simulink model "SoftRobot_AdaptivePassivity_FaultObserver_Regulation_S2"  (R2021b)
settings: Solver=FixedStepAuto  StartTime=0.0  StopTime=15  FixedStep=0.001  RelTol=1e-3  EnableMultiTasking=on
(part 1 of 2)
settings Model: Creator=Amirhosein  LastModifiedBy=sinar
settings SolverCC: AlgebraicLoopSolver=TrustRegion
settings DataIOCC: LimitDataPoints=on  SaveFormat=Array  ReturnWorkspaceOutputs=off
settings OptimizationCC: LifeSpan=inf
settings DebuggingCC: SFUnexpectedBacktrackingDiag=warning  SFNoUnconditionalDefaultTransitionDiag=warning  SFExecutionAtInitializationDiag=none  SFMachineParentedDataDiag=warning  ArithmeticOperatorsInVariantConditions=warning
settings HardwareCC: ProdBitPerPointer=32  ProdBitPerSizeT=32  ProdBitPerPtrDiffT=32  ProdLargestAtomicFloat=None  ProdIntDivRoundTo=Undefined  ProdEndianess=Unspecified  ProdWordSize=32  ProdHWDeviceType=32-bit Generic
settings ModelReferenceCC: PropagateSignalLabelsOutOfModel=off
settings SFSimCC: SimUseLocalCustomCode=off  CustomCodeUndefinedFunction=UseInterfaceOnly
settings RTWCC: RTWUseLocalCustomCode=off
settings CodeAppCC: StateflowObjectComments=on
settings GRTTargetCC: TargetLangStandard=C89/C90 (ANSI)
settings ConfigComp: CovMetricSettings=dw  CovSaveCumulativeToWorkspaceVar=on  CovSaveSingleToWorkspaceVar=on  CovExternalEMLEnable=off

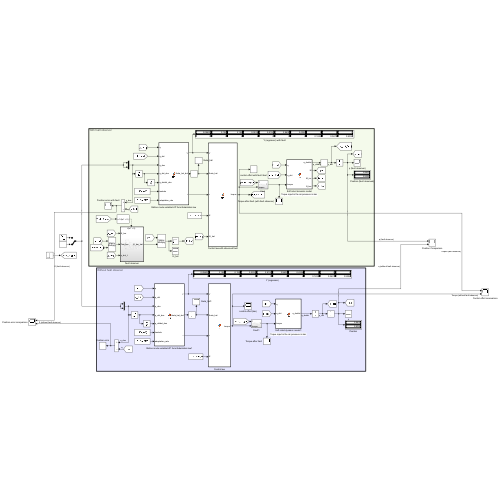
[thumbnail: Simulink's stored preview of the top-level diagram]
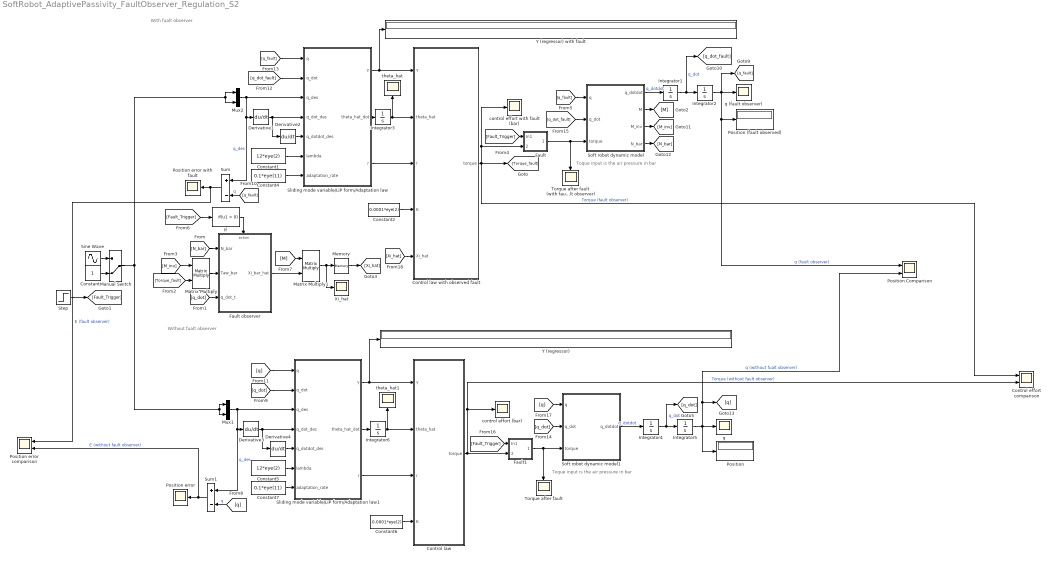
== system SoftRobot_AdaptivePassivity_FaultObserver_Regulation_S2 ==
  note: With fualt observer
  note: Without fualt observer
  note: Toque input is the air pressure in bar
  note: Toque input is the air pressure in bar
  Constant : Constant
  Constant1 : Constant  Value=12*eye(2)
  Constant2 : Constant  Value=0.0001*eye(2)
  Constant4 : Constant  Value=0.1*eye(11)
  Constant5 : Constant  Value=12*eye(2)
  Constant6 : Constant  Value=0.0001*eye(2)
  Constant7 : Constant  Value=0.1*eye(11)
  Control effort comparison : Scope  NumInputPorts=2
  Control law : MATLAB Function  TreatAsAtomicUnit=on
  Control law with observed fault : MATLAB Function  TreatAsAtomicUnit=on
  Derivative{1..4} (4 alike) : Derivative
  Fault : Subsystem
  Fault observer : Subsystem  TreatAsAtomicUnit=on
  Fault1 : Subsystem
  If : If  ShowElse=off
  Integrator1 : Integrator  InitialCondition=[0;0]
  Integrator2 : Integrator  InitialCondition=[0.1;0.1]
  Integrator3 : Integrator  InitialCondition=zeros(11,1)
  Integrator4 : Integrator  InitialCondition=[0;0]
  Integrator5 : Integrator  InitialCondition=[0.1;0.1]
  Integrator6 : Integrator  InitialCondition=zeros(11,1)
  Manual Switch : ManualSwitch  CurrentSetting=0
  Matrix Multiply : Product  Multiplication=Matrix(*)
  Matrix Multiply1 : Product  Multiplication=Matrix(*)
  Memory : Memory
  Mux1 : Mux  Inputs=2
  Mux2 : Mux  Inputs=2
  Position : Display
  Position (fault observed) : Display
  Position Comparison : Scope  NumInputPorts=2
  Position error : Scope
  Position error comparison : Scope  NumInputPorts=2
  Position error with fault : Scope
  Sine Wave : Sin  Amplitude=0.4  Bias=1  SampleTime=0
  Sliding mode variable/LIP form/Adaptation law : MATLAB Function  TreatAsAtomicUnit=on
  Sliding mode variable/LIP form/Adaptation law1 : MATLAB Function  TreatAsAtomicUnit=on
  Soft robot dynamic model : MATLAB Function  TreatAsAtomicUnit=on
  Soft robot dynamic model1 : MATLAB Function  TreatAsAtomicUnit=on
  Step : Step  Time=5  After=0.2  SampleTime=0
  Sum : Sum  Inputs=+-
  Sum1 : Sum  Inputs=+-
  Torque after fault : Scope
  Torque after fault (with fault observer) : Scope
  Xi_hat : Scope
  Y (regressor) : Display
  Y (regressor) with fault : Display
  control effort (bar) : Scope
  control effort with fault (bar) : Scope
  q : Scope
  q (fault observer) : Scope
  theta_hat : Scope
  theta_hat1 : Scope
  wires:
  Integrator2/1 -> Position Comparison/1, Position (fault observed)/1, [q_fault], q (fault observer)/1  "q (fault observer)"
  [q_dot_fault] -> Soft robot dynamic model/2(q_dot)
  [q_fault] -> Soft robot dynamic model/1(q)
  Sum/1 -> Position error comparison/1, Position error with fault/1  "E (fault observer)"
  Sliding mode variable/LIP form/Adaptation law/2(theta_hat_dot) -> Integrator3/1
  Soft robot dynamic model/1(q_dotdot) -> Integrator1/1  "q_dotdot"
  Integrator1/1 -> Integrator2/1, [q_dot_fault]  "q_dot"
  Control law with observed fault/1(torque) -> control effort with fault (bar)/1, Fault/2(torque), Control effort comparison/1, [Torque_fault]  "Torque (fault observer)"
  Constant1/1 -> Sliding mode variable/LIP form/Adaptation law/6(lambda)
  Constant4/1 -> Sliding mode variable/LIP form/Adaptation law/7(adaptation_rate)
  [q_dot_fault] -> Sliding mode variable/LIP form/Adaptation law/2(q_dot)
  [q_fault] -> Sliding mode variable/LIP form/Adaptation law/1(q)
  Mux2/1 -> Sum/1, Derivative1/1, Sliding mode variable/LIP form/Adaptation law/3(q_des)  "q_des"
  Derivative1/1 -> Derivative2/1, Sliding mode variable/LIP form/Adaptation law/4(q_dot_des)
  Derivative2/1 -> Sliding mode variable/LIP form/Adaptation law/5(q_dotdot_des)
  Sliding mode variable/LIP form/Adaptation law/1(Y) -> Y (regressor) with fault/1, Control law with observed fault/1(Y)
  Sliding mode variable/LIP form/Adaptation law/3(r) -> Control law with observed fault/3(r)
  Constant2/1 -> Control law with observed fault/4(K)
  [q_fault] -> Sum/2  "q"
  Manual Switch/1 -> Mux1/1, Mux1/2, Mux2/2, Mux2/1
  Fault/1(Out1) -> Soft robot dynamic model/3(torque), Torque after fault (with fault observer)/1
  Soft robot dynamic model/3(M_inv) -> [M_inv]
  Soft robot dynamic model/4(N_bar) -> [N_bar]
  [N_bar] -> Fault observer/1(N_bar)
  [M_inv] -> Matrix Multiply/1
  Matrix Multiply/1 -> Fault observer/2(Taw_bar)
  If/1 -> Fault observer/Action
  Step/1 -> [Fault_Trigger]
  [Fault_Trigger] -> If/1
  [q_dot] -> Fault observer/3(q_dot_t)
  Fault observer/1(Xi_bar_hat) -> Matrix Multiply1/2
  [Torque_fault] -> Matrix Multiply/2
  [Fault_Trigger] -> Fault/1(In1)
  Soft robot dynamic model/2(M) -> [M]
  [M] -> Matrix Multiply1/1
  Matrix Multiply1/1 -> Xi_hat/1, Memory/1
  [q] -> Sliding mode variable/LIP form/Adaptation law1/1(q)
  Constant7/1 -> Sliding mode variable/LIP form/Adaptation law1/7(adaptation_rate)
  Derivative3/1 -> Derivative4/1, Sliding mode variable/LIP form/Adaptation law1/4(q_dot_des)
  [Fault_Trigger] -> Fault1/1(In1)
  Constant5/1 -> Sliding mode variable/LIP form/Adaptation law1/6(lambda)
  Soft robot dynamic model1/1(q_dotdot) -> Integrator4/1  "q_dotdot"
  [q] -> Sum1/2  "q"
  Constant6/1 -> Control law/4(K)
  Sliding mode variable/LIP form/Adaptation law1/3(r) -> Control law/3(r)
  Integrator6/1 -> Control law/2(theta_hat), theta_hat1/1
  [q_dot] -> Soft robot dynamic model1/2(q_dot)
  Sliding mode variable/LIP form/Adaptation law1/2(theta_hat_dot) -> Integrator6/1
  Sliding mode variable/LIP form/Adaptation law1/1(Y) -> Y (regressor)/1, Control law/1(Y)
  Derivative4/1 -> Sliding mode variable/LIP form/Adaptation law1/5(q_dotdot_des)
  [q] -> Soft robot dynamic model1/1(q)
  Integrator4/1 -> Integrator5/1, [q_dot]  "q_dot"
  Mux1/1 -> Sum1/1, Derivative3/1, Sliding mode variable/LIP form/Adaptation law1/3(q_des)  "q_des"
  Integrator5/1 -> Position/1, Position Comparison/2, [q], q/1  "q (without fualt observer)"
  Control law/1(torque) -> Fault1/2(torque), control effort (bar)/1, Control effort comparison/2  "Torque (without fault observer)"
  Sum1/1 -> Position error comparison/2, Position error/1  "E (without fault observer)"
  Fault1/1(Out1) -> Soft robot dynamic model1/3(torque), Torque after fault/1
  [q_dot] -> Sliding mode variable/LIP form/Adaptation law1/2(q_dot)
  Memory/1 -> [Xi_hat]
  [Xi_hat] -> Control law with observed fault/5(Xi_hat)
  Integrator3/1 -> Control law with observed fault/2(theta_hat), theta_hat/1
  Sine Wave/1 -> Manual Switch/1
  Constant/1 -> Manual Switch/2

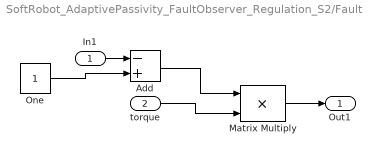
== system SoftRobot_AdaptivePassivity_FaultObserver_Regulation_S2/Fault ==
  In1 : Inport
  torque : Inport  Port=2
  Add : Sum  Inputs=-+
  Matrix Multiply : Product
  One : Constant  OutDataTypeStr=Inherit: Inherit via back propagation
  Out1 : Outport
  wires:
  In1/1 -> Add/1
  One/1 -> Add/2
  Matrix Multiply/1 -> Out1/1
  torque/1 -> Matrix Multiply/2
  Add/1 -> Matrix Multiply/1

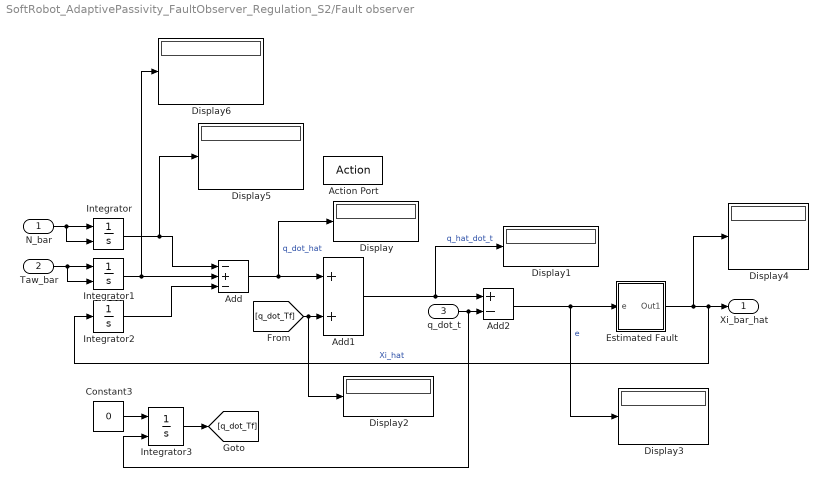
== system SoftRobot_AdaptivePassivity_FaultObserver_Regulation_S2/Fault observer ==
  N_bar : Inport
  Taw_bar : Inport  Port=2
  q_dot_t : Inport  Port=3
  Action Port : ActionPort  ActionPortLabel=if(u1 > 0)
  Add : Sum  Inputs=-+-
  Add1 : Sum
  Add2 : Sum  Inputs=+-
  Constant3 : Constant  Value=0
  Display{,1..6} (7 alike) : Display
  Estimated Fault : Subsystem
  Integrator : Integrator  InitialConditionSource=external
  Integrator1 : Integrator  InitialConditionSource=external
  Integrator2 : Integrator
  Integrator3 : Integrator  InitialConditionSource=external
  Xi_bar_hat : Outport
  wires:
  Integrator2/1 -> Add/3
  Estimated Fault/1(Out1) -> Display4/1, Integrator2/1, Xi_bar_hat/1  "Xi_hat"
  Add/1 -> Display/1, Add1/1  "q_dot_hat"
  Taw_bar/1 -> Integrator1/2, Integrator1/1
  Integrator/1 -> Display5/1, Add/1
  N_bar/1 -> Integrator/2, Integrator/1
  [q_dot_Tf] -> Display2/1, Add1/2
  Add1/1 -> Display1/1, Add2/1  "q_hat_dot_t"
  Add2/1 -> Display3/1, Estimated Fault/1(e)  "e"
  q_dot_t/1 -> Integrator3/2, Add2/2
  Integrator3/1 -> [q_dot_Tf]
  Constant3/1 -> Integrator3/1
  Integrator1/1 -> Display6/1, Add/2

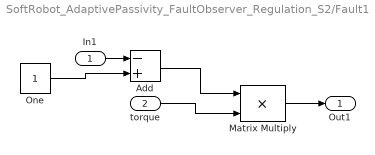
== system SoftRobot_AdaptivePassivity_FaultObserver_Regulation_S2/Fault1 ==
  In1 : Inport
  torque : Inport  Port=2
  Add : Sum  Inputs=-+
  Matrix Multiply : Product
  One : Constant  OutDataTypeStr=Inherit: Inherit via back propagation
  Out1 : Outport
  wires:
  In1/1 -> Add/1
  One/1 -> Add/2
  Matrix Multiply/1 -> Out1/1
  torque/1 -> Matrix Multiply/2
  Add/1 -> Matrix Multiply/1

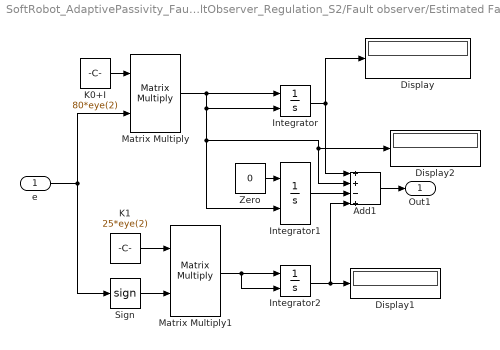
== system SoftRobot_AdaptivePassivity_FaultObserver_Regulation_S2/Fault observer/Estimated Fault ==
  e : Inport
  Add1 : Sum  Inputs=++-+
  Display : Display
  Display1 : Display
  Display2 : Display
  Integrator : Integrator  InitialConditionSource=external
  Integrator1 : Integrator  InitialConditionSource=external
  Integrator2 : Integrator  InitialConditionSource=external
  K0+I : Constant  Value=80*eye(2)
  K1 : Constant  Value=25*eye(2)
  Matrix Multiply : Product  Multiplication=Matrix(*)
  Matrix Multiply1 : Product  Multiplication=Matrix(*)
  Sign : Signum
  Zero : Constant  Value=0  OutDataTypeStr=Inherit: Inherit via back propagation
  Out1 : Outport
  wires:
  K0+I/1 -> Matrix Multiply/1
  K1/1 -> Matrix Multiply1/1
  Sign/1 -> Matrix Multiply1/2
  Add1/1 -> Out1/1
  Integrator/1 -> Display/1, Add1/1
  Matrix Multiply/1 -> Integrator/1, Integrator/2, Display2/1, Add1/2, Integrator1/2
  e/1 -> Sign/1, Matrix Multiply/2
  Matrix Multiply1/1 -> Integrator2/2, Integrator2/1
  Integrator1/1 -> Add1/3
  Integrator2/1 -> Display1/1, Add1/4
  Zero/1 -> Integrator1/1

== matlab function SoftRobot_AdaptivePassivity_FaultObserver_Regulation_S2/Control law ==
  data: Y input; theta_hat input; r input; torque output; K input
function torque = fcn(Y,theta_hat,r,K)

torque = Y*theta_hat-K*r;

== matlab function SoftRobot_AdaptivePassivity_FaultObserver_Regulation_S2/Sliding mode variable//LIP form//Adaptation law1 ==
  data: Y output; q input; q_dot input; q_des input; theta_hat_dot output; q_dot_des input; q_dotdot_des input; lambda input; adaptation_rate input; r output
function [Y,theta_hat_dot,r] = fcn(q,q_dot,q_des,q_dot_des,q_dotdot_des,lambda,adaptation_rate)

l1=0.067;
l2=0.077;

q1 = q(1);
q2 = q(2);
q_dot1 = q_dot(1);
q_dot2 = q_dot(2);

v = q_dot_des-lambda*(q-q_des);
v1 = v(1);
v2 = v(2);

v_dot = q_dotdot_des-lambda*(q_dot-q_dot_des);
v_dot1 = v_dot(1);
v_dot2 = v_dot(2);

Y1 = [((981*l1*q2*sin(q1))/200 - (981*l1*q1*q2*cos(q1))/200)/(q1^2*q2) - v1*((q_dot2*((2*((l1^2*q2^2)/2 + (l1^2*q1^2*q2^2)/4 - (l1^2*q2^2*cos(q1))/2 - (l1^2*q1*q2^2*sin(q1))/2))/(q1^4*q2^3) - (l1^2*q2 + (l1^2*q1^2*q2)/2 - l1^2*q2*cos(q1) - l1^2*q1*q2*sin(q1))/(q1^4*q2^2)))/2 - (q_dot1*(((l1^2*q1*q2^2)/2 - (l1^2*q1*q2^2*cos(q1))/2)/(q1^4*q2^2) - (4*((l1^2*q2^2)/2 + (l1^2*q1^2*q2^2)/4 - (l1^2*q2^2*cos(q1))/2 - (l1^2*q1*q2^2*sin(q1))/2))/(q1^5*q2^2)))/2) + (v_dot1*((l1^2*q2^2)/2 + (l1^2*q1^2*q2^2)/4 - (l1^2*q2^2*cos(q1))/2 - (l1^2*q1*q2^2*sin(q1))/2))/(q1^4*q2^2), ((981*l1*q2*sin(q1))/100 - (981*l1*q1*q2*cos(q1))/100)/(q1^2*q2) - v1*((q_dot2*((2*(2*l1^2*q2^2 + l1^2*q1^2*q2^2 - 2*l1^2*q2^2*cos(q1) - 2*l1^2*q1*q2^2*sin(q1)))/(q1^4*q2^3) - (4*l1^2*q2 + 2*l1^2*q1^2*q2 - 4*l1^2*q2*cos(q1) - 4*l1^2*q1*q2*sin(q1))/(q1^4*q2^2)))/2 - (q_dot1*((2*l1^2*q1*q2^2 - 2*l1^2*q1*q2^2*cos(q1))/(q1^4*q2^2) - (4*(2*l1^2*q2^2 + l1^2*q1^2*q2^2 - 2*l1^2*q2^2*cos(q1) - 2*l1^2*q1*q2^2*sin(q1)))/(q1^5*q2^2)))/2) + (v_dot1*(2*l1^2*q2^2 + l1^2*q1^2*q2^2 - 2*l1^2*q2^2*cos(q1) - 2*l1^2*q1*q2^2*sin(q1)))/(q1^4*q2^2), ((981*l1*q2*sin(q1))/100 - (981*l1*q1*q2*cos(q1))/100)/(q1^2*q2) - v1*((q_dot2*((2*(2*l1^2*q2^2 + l1^2*q1^2*q2^2 - 2*l1^2*q2^2*cos(q1) - 2*l1^2*q1*q2^2*sin(q1)))/(q1^4*q2^3) - (4*l1^2*q2 + 2*l1^2*q1^2*q2 - 4*l1^2*q2*cos(q1) - 4*l1^2*q1*q2*sin(q1))/(q1^4*q2^2)))/2 - (q_dot1*((2*l1^2*q1*q2^2 - 2*l1^2*q1*q2^2*cos(q1))/(q1^4*q2^2) - (4*(2*l1^2*q2^2 + l1^2*q1^2*q2^2 - 2*l1^2*q2^2*cos(q1) - 2*l1^2*q1*q2^2*sin(q1)))/(q1^5*q2^2)))/2) + (v_dot1*(2*l1^2*q2^2 + l1^2*q1^2*q2^2 - 2*l1^2*q2^2*cos(q1) - 2*l1^2*q1*q2^2*sin(q1)))/(q1^4*q2^2), ((981*l1*q2*sin(q1))/100 - (981*l2*q1^2*cos(q1 + q2))/200 + (981*l2*q1^2*cos(q1))/200 - (981*l1*q1*q2*cos(q1))/100)/(q1^2*q2) - v1*((q_dot1*((4*(2*l1^2*q2^2 + (l2^2*q1^4)/2 + l1^2*q1^2*q2^2 - 2*l1^2*q2^2*cos(q1) - (l2^2*q1^4*cos(q2))/2 - 2*l1^2*q1*q2^2*sin(q1) - l1*l2*q1^3*q2 - l1*l2*q1^2*q2*sin(q1 + q2) + l1*l2*q1^3*q2*cos(q2) + l1*l2*q1^2*q2*sin(q1) + l1*l2*q1^2*q2*sin(q2)))/(q1^5*q2^2) - (2*l2^2*q1^3 + 2*l1^2*q1*q2^2 - 2*l2^2*q1^3*cos(q2) - 2*l1^2*q1*q2^2*cos(q1) - 3*l1*l2*q1^2*q2 - l1*l2*q1^2*q2*cos(q1 + q2) + l1*l2*q1^2*q2*cos(q1) + 3*l1*l2*q1^2*q2*cos(q2) - 2*l1*l2*q1*q2*sin(q1 + q2) + 2*l1*l2*q1*q2*sin(q1) + 2*l1*l2*q1*q2*sin(q2))/(q1^4*q2^2)))/2 + (q_dot2*((2*(2*l1^2*q2^2 + (l2^2*q1^4)/2 + l1^2*q1^2*q2^2 - 2*l1^2*q2^2*cos(q1) - (l2^2*q1^4*cos(q2))/2 - 2*l1^2*q1*q2^2*sin(q1) - l1*l2*q1^3*q2 - l1*l2*q1^2*q2*sin(q1 + q2) + l1*l2*q1^3*q2*cos(q2) + l1*l2*q1^2*q2*sin(q1) + l1*l2*q1^2*q2*sin(q2)))/(q1^4*q2^3) - (4*l1^2*q2 - l1*l2*q1^3 + 2*l1^2*q1^2*q2 - 4*l1^2*q2*cos(q1) + (l2^2*q1^4*sin(q2))/2 - l1*l2*q1^2*sin(q1 + q2) + l1*l2*q1^3*cos(q2) + l1*l2*q1^2*sin(q1) + l1*l2*q1^2*sin(q2) - 4*l1^2*q1*q2*sin(q1) - l1*l2*q1^2*q2*cos(q1 + q2) + l1*l2*q1^2*q2*cos(q2) - l1*l2*q1^3*q2*sin(q2))/(q1^4*q2^2)))/2) + (v_dot1*(2*l1^2*q2^2 + (l2^2*q1^4)/2 + l1^2*q1^2*q2^2 - 2*l1^2*q2^2*cos(q1) - (l2^2*q1^4*cos(q2))/2 - 2*l1^2*q1*q2^2*sin(q1) - l1*l2*q1^3*q2 - l1*l2*q1^2*q2*sin(q1 + q2) + l1*l2*q1^3*q2*cos(q2) + l1*l2*q1^2*q2*sin(q1) + l1*l2*q1^2*q2*sin(q2)))/(q1^4*q2^2) - (l2*v2*(2*l2*q1^2*q_dot1 - 4*l1*q_dot2 + 2*l2*q1^2*q_dot2 + 4*l1*q_dot2*cos(q1) + 4*l1*q_dot2*cos(q2) - 4*l1*q_dot2*cos(q1 + q2) - 2*l1*q1*q2*q_dot1 - 2*l1*q2*q_dot1*sin(q1 + q2) - 4*l1*q2*q_dot2*sin(q1 + q2) + 2*l1*q2*q_dot1*sin(q1) - 4*l1*q1*q_dot2*sin(q2) + 2*l1*q2*q_dot1*sin(q2) + 4*l1*q2*q_dot2*sin(q2) + 2*l1*q2^2*q_dot1*cos(q1 + q2) + 2*l1*q2^2*q_dot2*cos(q1 + q2) - 2*l1*q2^2*q_dot1*cos(q2) - 2*l2*q1^2*q_dot1*cos(q2) - 2*l1*q2^2*q_dot2*cos(q2) - 2*l2*q1^2*q_dot2*cos(q2) + 2*l1*q1*q2^2*q_dot1*sin(q2) + 2*l1*q1*q2^2*q_dot2*sin(q2) - l2*q1^2*q2*q_dot1*sin(q2) - l2*q1^2*q2*q_dot2*sin(q2) + 2*l1*q1*q2*q_dot1*cos(q2) + 4*l1*q1*q2*q_dot2*cos(q2)))/(4*q1^2*q2^3) - (l2*v_dot2*(2*l1 + 2*l1*cos(q1 + q2) - l2*q1^2 - 2*l1*cos(q1) - 2*l1*cos(q2) + 2*l1*q1*sin(q2) - 2*l1*q2*sin(q2) + l2*q1^2*cos(q2) + 2*l1*q2*sin(q1 + q2) - 2*l1*q1*q2*cos(q2)))/(4*q1^2*q2^2), ((981*l1*q2*sin(q1))/100 - (981*l2*q1^2*cos(q1 + q2))/100 + (981*l2*q1^2*cos(q1))/100 - (981*l1*q1*q2*cos(q1))/100)/(q1^2*q2) - v1*((q_dot1*((4*(2*l1^2*q2^2 + 2*l2^2*q1^4 + l1^2*q1^2*q2^2 - 2*l1^2*q2^2*cos(q1) - 2*l2^2*q1^4*cos(q2) - 2*l1^2*q1*q2^2*sin(q1) - 2*l1*l2*q1^3*q2 - 2*l1*l2*q1^2*q2*sin(q1 + q2) + 2*l1*l2*q1^3*q2*cos(q2) + 2*l1*l2*q1^2*q2*sin(q1) + 2*l1*l2*q1^2*q2*sin(q2)))/(q1^5*q2^2) - (8*l2^2*q1^3 + 2*l1^2*q1*q2^2 - 8*l2^2*q1^3*cos(q2) - 2*l1^2*q1*q2^2*cos(q1) - 6*l1*l2*q1^2*q2 - 2*l1*l2*q1^2*q2*cos(q1 + q2) + 2*l1*l2*q1^2*q2*cos(q1) + 6*l1*l2*q1^2*q2*cos(q2) - 4*l1*l2*q1*q2*sin(q1 + q2) + 4*l1*l2*q1*q2*sin(q1) + 4*l1*l2*q1*q2*sin(q2))/(q1^4*q2^2)))/2 + (q_dot2*((2*(2*l1^2*q2^2 + 2*l2^2*q1^4 + l1^2*q1^2*q2^2 - 2*l1^2*q2^2*cos(q1) - 2*l2^2*q1^4*cos(q2) - 2*l1^2*q1*q2^2*sin(q1) - 2*l1*l2*q1^3*q2 - 2*l1*l2*q1^2*q2*sin(q1 + q2) + 2*l1*l2*q1^3*q2*cos(q2) + 2*l1*l2*q1^2*q2*sin(q1) + 2*l1*l2*q1^2*q2*sin(q2)))/(q1^4*q2^3) - (4*l1^2*q2 - 2*l1*l2*q1^3 + 2*l1^2*q1^2*q2 - 4*l1^2*q2*cos(q1) + 2*l2^2*q1^4*sin(q2) - 2*l1*l2*q1^2*sin(q1 + q2) + 2*l1*l2*q1^3*cos(q2) + 2*l1*l2*q1^2*sin(q1) + 2*l1*l2*q1^2*sin(q2) - 4*l1^2*q1*q2*sin(q1) - 2*l1*l2*q1^2*q2*cos(q1 + q2) + 2*l1*l2*q1^2*q2*cos(q2) - 2*l1*l2*q1^3*q2*sin(q2))/(q1^4*q2^2)))/2) + (v_dot1*(2*l1^2*q2^2 + 2*l2^2*q1^4 + l1^2*q1^2*q2^2 - 2*l1^2*q2^2*cos(q1) - 2*l2^2*q1^4*cos(q2) - 2*l1^2*q1*q2^2*sin(q1) - 2*l1*l2*q1^3*q2 - 2*l1*l2*q1^2*q2*sin(q1 + q2) + 2*l1*l2*q1^3*q2*cos(q2) + 2*l1*l2*q1^2*q2*sin(q1) + 2*l1*l2*q1^2*q2*sin(q2)))/(q1^4*q2^2) - (l2*v2*(8*l2*q1^2*q_dot1 - 8*l1*q_dot2 + 8*l2*q1^2*q_dot2 + 8*l1*q_dot2*cos(q1) + 8*l1*q_dot2*cos(q2) - 8*l1*q_dot2*cos(q1 + q2) - 4*l1*q1*q2*q_dot1 - 4*l1*q2*q_dot1*sin(q1 + q2) - 8*l1*q2*q_dot2*sin(q1 + q2) + 4*l1*q2*q_dot1*sin(q1) - 8*l1*q1*q_dot2*sin(q2) + 4*l1*q2*q_dot1*sin(q2) + 8*l1*q2*q_dot2*sin(q2) + 4*l1*q2^2*q_dot1*cos(q1 + q2) + 4*l1*q2^2*q_dot2*cos(q1 + q2) - 4*l1*q2^2*q_dot1*cos(q2) - 8*l2*q1^2*q_dot1*cos(q2) - 4*l1*q2^2*q_dot2*cos(q2) - 8*l2*q1^2*q_dot2*cos(q2) + 4*l1*q1*q2^2*q_dot1*sin(q2) + 4*l1*q1*q2^2*q_dot2*sin(q2) - 4*l2*q1^2*q2*q_dot1*sin(q2) - 4*l2*q1^2*q2*q_dot2*sin(q2) + 4*l1*q1*q2*q_dot1*cos(q2) + 8*l1*q1*q2*q_dot2*cos(q2)))/(4*q1^2*q2^3) - (l2*v_dot2*(4*l1 + 4*l1*cos(q1 + q2) - 4*l2*q1^2 - 4*l1*cos(q1) - 4*l1*cos(q2) + 4*l1*q1*sin(q2) - 4*l1*q2*sin(q2) + 4*l2*q1^2*cos(q2) + 4*l1*q2*sin(q1 + q2) - 4*l1*q1*q2*cos(q2)))/(4*q1^2*q2^2), q1, v1];
Y2 = [(q_dot2*v2*((l2^2*(2*cos(q2) + 2*q2*sin(q2) - q2^2 - 2))/q2^5 + (l2^2*(2*q2 - 2*q2*cos(q2)))/(4*q2^4)))/2 - (981*l2*(sin(q1) - sin(q1 + q2) + q2*cos(q1 + q2)))/(200*q2^2) - (l2^2*v_dot2*(2*cos(q2) + 2*q2*sin(q2) - q2^2 - 2))/(4*q2^4) - (l2*v_dot1*(2*l1 + 2*l1*cos(q1 + q2) - l2*q1^2 - 2*l1*cos(q1) - 2*l1*cos(q2) + 2*l1*q1*sin(q2) - 2*l1*q2*sin(q2) + l2*q1^2*cos(q2) + 2*l1*q2*sin(q1 + q2) - 2*l1*q1*q2*cos(q2)))/(4*q1^2*q2^2) + (l2*q_dot1*v1*(4*l1*q2 + 2*l2*q1^3 - 2*l1*q1^2*q2 - 4*l1*q2*cos(q1) - 4*l1*q2*cos(q2) + 4*l1*q2^2*sin(q1 + q2) - 2*l2*q1^3*cos(q2) - 4*l1*q2^2*sin(q2) + 4*l1*q2*cos(q1 + q2) + 2*l1*q1^2*q2^2*sin(q2) + 4*l1*q1*q2*sin(q2) - 4*l1*q1*q2^2*cos(q2) + 2*l1*q1^2*q2*cos(q2) - l2*q1^3*q2*sin(q2)))/(4*q1^3*q2^3), (q_dot2*v2*((4*l2^2*(2*cos(q2) + 2*q2*sin(q2) - q2^2 - 2))/q2^5 + (l2^2*(2*q2 - 2*q2*cos(q2)))/q2^4))/2 - (981*l2*(sin(q1) - sin(q1 + q2) + q2*cos(q1 + q2)))/(100*q2^2) - (l2^2*v_dot2*(2*cos(q2) + 2*q2*sin(q2) - q2^2 - 2))/q2^4 - (l2*v_dot1*(4*l1 + 4*l1*cos(q1 + q2) - 4*l2*q1^2 - 4*l1*cos(q1) - 4*l1*cos(q2) + 4*l1*q1*sin(q2) - 4*l1*q2*sin(q2) + 4*l2*q1^2*cos(q2) + 4*l1*q2*sin(q1 + q2) - 4*l1*q1*q2*cos(q2)))/(4*q1^2*q2^2) + (l2*q_dot1*v1*(8*l1*q2 + 8*l2*q1^3 - 4*l1*q1^2*q2 - 8*l1*q2*cos(q1) - 8*l1*q2*cos(q2) + 8*l1*q2^2*sin(q1 + q2) - 8*l2*q1^3*cos(q2) - 8*l1*q2^2*sin(q2) + 8*l1*q2*cos(q1 + q2) + 4*l1*q1^2*q2^2*sin(q2) + 8*l1*q1*q2*sin(q2) - 8*l1*q1*q2^2*cos(q2) + 4*l1*q1^2*q2*cos(q2) - 4*l2*q1^3*q2*sin(q2)))/(4*q1^3*q2^3), q2, v2];
Y = blkdiag(Y1,Y2);

% Y=[ -(l1*(981*q1^4*cos(q1) - 981*q1^3*sin(q1) - 50*l1*q1^3*v_dot1 - 100*l1*q1*v_dot1 + 200*l1*q_dot1*v1 + 50*l1*q1^2*q_dot1*v1 + 100*l1*q1*v_dot1*cos(q1) - 200*l1*q_dot1*v1*cos(q1) + 100*l1*q1^2*v_dot1*sin(q1) - 200*l1*q1*q_dot1*v1*sin(q1) + 50*l1*q1^2*q_dot1*v1*cos(q1)))/(200*q1^5), -(l1*(981*q1^4*cos(q1) - 981*q1^3*sin(q1) - 100*l1*q1^3*v_dot1 - 200*l1*q1*v_dot1 + 400*l1*q_dot1*v1 + 100*l1*q1^2*q_dot1*v1 + 200*l1*q1*v_dot1*cos(q1) - 400*l1*q_dot1*v1*cos(q1) + 200*l1*q1^2*v_dot1*sin(q1) - 400*l1*q1*q_dot1*v1*sin(q1) + 100*l1*q1^2*q_dot1*v1*cos(q1)))/(100*q1^5), -(l1*(981*q1^4*cos(q1) - 981*q1^3*sin(q1) - 100*l1*q1^3*v_dot1 - 200*l1*q1*v_dot1 + 400*l1*q_dot1*v1 + 100*l1*q1^2*q_dot1*v1 + 200*l1*q1*v_dot1*cos(q1) - 400*l1*q_dot1*v1*cos(q1) + 200*l1*q1^2*v_dot1*sin(q1) - 400*l1*q1*q_dot1*v1*sin(q1) + 100*l1*q1^2*q_dot1*v1*cos(q1)))/(100*q1^5), (1962*l1*q2*sin(q1) - 981*l2*q1^2*cos(q1 + q2) + 981*l2*q1^2*cos(q1) - 1962*l1*q1*q2*cos(q1))/(200*q1^2*q2) + (v_dot1*(2*l1^2*q2^2 + (l2^2*q1^4)/2 + l1^2*q1^2*q2^2 - 2*l1^2*q2^2*cos(q1) - (l2^2*q1^4*cos(q2))/2 - 2*l1^2*q1*q2^2*sin(q1) - l1*l2*q1^3*q2 - l1*l2*q1^2*q2*sin(q1 + q2) + l1*l2*q1^3*q2*cos(q2) + l1*l2*q1^2*q2*sin(q1) + l1*l2*q1^2*q2*sin(q2)))/(q1^4*q2^2) - (l2*v2*(4*l2*q1^2*q_dot1 - 4*l1*q_dot2 + 2*l2*q1^2*q_dot2 + 4*l1*q_dot2*cos(q1) + 4*l1*q_dot2*cos(q2) - 4*l1*q_dot2*cos(q1 + q2) - 4*l1*q1*q2*q_dot1 - 4*l1*q2*q_dot1*sin(q1 + q2) - 4*l1*q2*q_dot2*sin(q1 + q2) + 4*l1*q2*q_dot1*sin(q1) - 4*l1*q1*q_dot2*sin(q2) + 4*l1*q2*q_dot1*sin(q2) + 4*l1*q2*q_dot2*sin(q2) + 4*l1*q2^2*q_dot1*cos(q1 + q2) + 2*l1*q2^2*q_dot2*cos(q1 + q2) - 4*l1*q2^2*q_dot1*cos(q2) - 4*l2*q1^2*q_dot1*cos(q2) - 2*l1*q2^2*q_dot2*cos(q2) - 2*l2*q1^2*q_dot2*cos(q2) + 4*l1*q1*q2^2*q_dot1*sin(q2) + 2*l1*q1*q2^2*q_dot2*sin(q2) - 2*l2*q1^2*q2*q_dot1*sin(q2) - l2*q1^2*q2*q_dot2*sin(q2) + 4*l1*q1*q2*q_dot1*cos(q2) + 4*l1*q1*q2*q_dot2*cos(q2)))/(4*q1^2*q2^3) - (l2*v_dot2*(2*l1 + 2*l1*cos(q1 + q2) - l2*q1^2 - 2*l1*cos(q1) - 2*l1*cos(q2) + 2*l1*q1*sin(q2) - 2*l1*q2*sin(q2) + l2*q1^2*cos(q2) + 2*l1*q2*sin(q1 + q2) - 2*l1*q1*q2*cos(q2)))/(4*q1^2*q2^2) - (l1*q_dot1*v1*(8*l1*q2 - l2*q1^3 + 2*l1*q1^2*q2 - 8*l1*q2*cos(q1) + l2*q1^3*cos(q1 + q2) - 2*l2*q1^2*sin(q1 + q2) - l2*q1^3*cos(q1) + l2*q1^3*cos(q2) + 2*l2*q1^2*sin(q1) + 2*l2*q1^2*sin(q2) - 8*l1*q1*q2*sin(q1) + 2*l1*q1^2*q2*cos(q1)))/(2*q1^5*q2), (981*l1*q2*sin(q1) - 981*l2*q1^2*cos(q1 + q2) + 981*l2*q1^2*cos(q1) - 981*l1*q1*q2*cos(q1))/(100*q1^2*q2) + (v_dot1*(2*l1^2*q2^2 + 2*l2^2*q1^4 + l1^2*q1^2*q2^2 - 2*l1^2*q2^2*cos(q1) - 2*l2^2*q1^4*cos(q2) - 2*l1^2*q1*q2^2*sin(q1) - 2*l1*l2*q1^3*q2 - 2*l1*l2*q1^2*q2*sin(q1 + q2) + 2*l1*l2*q1^3*q2*cos(q2) + 2*l1*l2*q1^2*q2*sin(q1) + 2*l1*l2*q1^2*q2*sin(q2)))/(q1^4*q2^2) - (l2*v2*(4*l2*q1^2*q_dot1 - 2*l1*q_dot2 + 2*l2*q1^2*q_dot2 + 2*l1*q_dot2*cos(q1) + 2*l1*q_dot2*cos(q2) - 2*l1*q_dot2*cos(q1 + q2) - 2*l1*q1*q2*q_dot1 - 2*l1*q2*q_dot1*sin(q1 + q2) - 2*l1*q2*q_dot2*sin(q1 + q2) + 2*l1*q2*q_dot1*sin(q1) - 2*l1*q1*q_dot2*sin(q2) + 2*l1*q2*q_dot1*sin(q2) + 2*l1*q2*q_dot2*sin(q2) + 2*l1*q2^2*q_dot1*cos(q1 + q2) + l1*q2^2*q_dot2*cos(q1 + q2) - 2*l1*q2^2*q_dot1*cos(q2) - 4*l2*q1^2*q_dot1*cos(q2) - l1*q2^2*q_dot2*cos(q2) - 2*l2*q1^2*q_dot2*cos(q2) + 2*l1*q1*q2^2*q_dot1*sin(q2) + l1*q1*q2^2*q_dot2*sin(q2) - 2*l2*q1^2*q2*q_dot1*sin(q2) - l2*q1^2*q2*q_dot2*sin(q2) + 2*l1*q1*q2*q_dot1*cos(q2) + 2*l1*q1*q2*q_dot2*cos(q2)))/(q1^2*q2^3) - (l2*v_dot2*(4*l1 + 4*l1*cos(q1 + q2) - 4*l2*q1^2 - 4*l1*cos(q1) - 4*l1*cos(q2) + 4*l1*q1*sin(q2) - 4*l1*q2*sin(q2) + 4*l2*q1^2*cos(q2) + 4*l1*q2*sin(q1 + q2) - 4*l1*q1*q2*cos(q2)))/(4*q1^2*q2^2) - (l1*q_dot1*v1*(4*l1*q2 - l2*q1^3 + l1*q1^2*q2 - 4*l1*q2*cos(q1) + l2*q1^3*cos(q1 + q2) - 2*l2*q1^2*sin(q1 + q2) - l2*q1^3*cos(q1) + l2*q1^3*cos(q2) + 2*l2*q1^2*sin(q1) + 2*l2*q1^2*sin(q2) - 4*l1*q1*q2*sin(q1) + l1*q1^2*q2*cos(q1)))/(q1^5*q2), q1,  0, v1,      0
%                                                                                                                                                                                                                                                                                                                   0,                                                                                                                                                                                                                                                                                                                     0,                                                                                                                                                                                                                                                                                                                     0,                                                                                                                                                                                                                                                                                                                                                                                                                                                                                                                                                                                                                                                                                                                                                                                  (l2*q_dot1*v1*(4*l1*q2 + 2*l2*q1^3 - 2*l1*q1^2*q2 - 4*l1*q2*cos(q1) - 4*l1*q2*cos(q2) + 4*l1*q2^2*sin(q1 + q2) - 2*l2*q1^3*cos(q2) - 4*l1*q2^2*sin(q2) + 4*l1*q2*cos(q1 + q2) + 2*l1*q1^2*q2^2*sin(q2) + 4*l1*q1*q2*sin(q2) - 4*l1*q1*q2^2*cos(q2) + 2*l1*q1^2*q2*cos(q2) - l2*q1^3*q2*sin(q2)))/(4*q1^3*q2^3) - (l2^2*v_dot2*(2*cos(q2) + 2*q2*sin(q2) - q2^2 - 2))/(4*q2^4) - (l2*v_dot1*(2*l1 + 2*l1*cos(q1 + q2) - l2*q1^2 - 2*l1*cos(q1) - 2*l1*cos(q2) + 2*l1*q1*sin(q2) - 2*l1*q2*sin(q2) + l2*q1^2*cos(q2) + 2*l1*q2*sin(q1 + q2) - 2*l1*q1*q2*cos(q2)))/(4*q1^2*q2^2) - (l2^2*q_dot2*v2*(q2^2*cos(q2) - 4*cos(q2) - 4*q2*sin(q2) + q2^2 + 4))/(4*q2^5) - (981*l2*(sin(q1) - sin(q1 + q2) + q2*cos(q1 + q2)))/(200*q2^2),                                                                                                                                                                                                                                                                                                                                                                                                                                                                                                                                                                                                                                                                                                                                                                                        (l2*q_dot1*v1*(2*l1*q2 + 2*l2*q1^3 - l1*q1^2*q2 - 2*l1*q2*cos(q1) - 2*l1*q2*cos(q2) + 2*l1*q2^2*sin(q1 + q2) - 2*l2*q1^3*cos(q2) - 2*l1*q2^2*sin(q2) + 2*l1*q2*cos(q1 + q2) + l1*q1^2*q2^2*sin(q2) + 2*l1*q1*q2*sin(q2) - 2*l1*q1*q2^2*cos(q2) + l1*q1^2*q2*cos(q2) - l2*q1^3*q2*sin(q2)))/(q1^3*q2^3) - (l2^2*v_dot2*(2*cos(q2) + 2*q2*sin(q2) - q2^2 - 2))/q2^4 - (l2*v_dot1*(4*l1 + 4*l1*cos(q1 + q2) - 4*l2*q1^2 - 4*l1*cos(q1) - 4*l1*cos(q2) + 4*l1*q1*sin(q2) - 4*l1*q2*sin(q2) + 4*l2*q1^2*cos(q2) + 4*l1*q2*sin(q1 + q2) - 4*l1*q1*q2*cos(q2)))/(4*q1^2*q2^2) - (l2^2*q_dot2*v2*(q2^2*cos(q2) - 4*cos(q2) - 4*q2*sin(q2) + q2^2 + 4))/q2^5 - (981*l2*(sin(q1) - sin(q1 + q2) + q2*cos(q1 + q2)))/(100*q2^2),  0, q2,      0, v2];
% 
r = [q_dot1;q_dot2]-v;

theta_hat_dot = -adaptation_rate*Y'*r;

== matlab function SoftRobot_AdaptivePassivity_FaultObserver_Regulation_S2/Soft robot dynamic model1 ==
  data: q_dotdot output; q input; q_dot input; torque input
function q_dotdot  = fcn(q,q_dot,torque)

mu1 = 0.02/3;
mu2 = 0.02/3;
mu3 = 0;
mu4 = 0.02/3;
l1 = 0.067;
l2 = 0.077;
mu5 = 0.0251/3;
mu6 = 0.0251/3;
mu7 = 0;
mu8 = 0.0251/3;

q1 = q(1);
q2 = q(2);
qdot1 = q_dot(1);
qdot2 = q_dot(2);

M=[ (0.25*(2.0*l1^2*mu2*q2^2 + 8.0*l1^2*mu4*q2^2 + 8.0*l1^2*mu5*q2^2 + 8.0*l1^2*mu6*q2^2 + 8.0*l1^2*mu8*q2^2 + 2.0*l2^2*mu6*q1^4 + 8.0*l2^2*mu8*q1^4 + l1^2*mu2*q1^2*q2^2 + 4.0*l1^2*mu4*q1^2*q2^2 + 4.0*l1^2*mu5*q1^2*q2^2 + 4.0*l1^2*mu6*q1^2*q2^2 + 4.0*l1^2*mu8*q1^2*q2^2 - 2.0*l1^2*mu2*q2^2*cos(q1) - 8.0*l1^2*mu4*q2^2*cos(q1) - 8.0*l1^2*mu5*q2^2*cos(q1) - 8.0*l1^2*mu6*q2^2*cos(q1) - 8.0*l1^2*mu8*q2^2*cos(q1) - 2.0*l2^2*mu6*q1^4*cos(q2) - 8.0*l2^2*mu8*q1^4*cos(q2) - 2.0*l1^2*mu2*q1*q2^2*sin(q1) - 8.0*l1^2*mu4*q1*q2^2*sin(q1) - 8.0*l1^2*mu5*q1*q2^2*sin(q1) - 8.0*l1^2*mu6*q1*q2^2*sin(q1) - 8.0*l1^2*mu8*q1*q2^2*sin(q1) - 4.0*l1*l2*mu6*q1^3*q2 - 8.0*l1*l2*mu8*q1^3*q2 - 4.0*l1*l2*mu6*q1^2*q2*sin(q1 + q2) - 8.0*l1*l2*mu8*q1^2*q2*sin(q1 + q2) + 4.0*l1*l2*mu6*q1^3*q2*cos(q2) + 8.0*l1*l2*mu8*q1^3*q2*cos(q2) + 4.0*l1*l2*mu6*q1^2*q2*sin(q1) + 4.0*l1*l2*mu6*q1^2*q2*sin(q2) + 8.0*l1*l2*mu8*q1^2*q2*sin(q1) + 8.0*l1*l2*mu8*q1^2*q2*sin(q2)))/(q1^4*q2^2), -(0.25*l2*(2.0*l1*mu6 + 4.0*l1*mu8 - 1.0*l2*mu6*q1^2 - 4.0*l2*mu8*q1^2 - 2.0*l1*mu6*cos(q1) - 2.0*l1*mu6*cos(q2) - 4.0*l1*mu8*cos(q1) - 4.0*l1*mu8*cos(q2) + 2.0*l1*mu6*cos(q1 + q2) + 4.0*l1*mu8*cos(q1 + q2) + 2.0*l1*mu6*q2*sin(q1 + q2) + 4.0*l1*mu8*q2*sin(q1 + q2) + 2.0*l1*mu6*q1*sin(q2) - 2.0*l1*mu6*q2*sin(q2) + 4.0*l1*mu8*q1*sin(q2) - 4.0*l1*mu8*q2*sin(q2) + l2*mu6*q1^2*cos(q2) + 4.0*l2*mu8*q1^2*cos(q2) - 2.0*l1*mu6*q1*q2*cos(q2) - 4.0*l1*mu8*q1*q2*cos(q2)))/(q1^2*q2^2)
                                                                                                                                                                                                                                                                                                                                                                                                                                                                                     -(0.25*l2*(2.0*l1*mu6 + 4.0*l1*mu8 - 1.0*l2*mu6*q1^2 - 4.0*l2*mu8*q1^2 - 2.0*l1*mu6*cos(q1) - 2.0*l1*mu6*cos(q2) - 4.0*l1*mu8*cos(q1) - 4.0*l1*mu8*cos(q2) + 2.0*l1*mu6*cos(q1 + q2) + 4.0*l1*mu8*cos(q1 + q2) + 2.0*l1*mu6*q2*sin(q1 + q2) + 4.0*l1*mu8*q2*sin(q1 + q2) + 2.0*l1*mu6*q1*sin(q2) - 2.0*l1*mu6*q2*sin(q2) + 4.0*l1*mu8*q1*sin(q2) - 4.0*l1*mu8*q2*sin(q2) + l2*mu6*q1^2*cos(q2) + 4.0*l2*mu8*q1^2*cos(q2) - 2.0*l1*mu6*q1*q2*cos(q2) - 4.0*l1*mu8*q1*q2*cos(q2)))/(q1^2*q2^2),                                                                                                                                                                                                                                                                                                                                                                                                            -(0.25*l2^2*(mu6 + 4.0*mu8)*(2.0*cos(q2) + 2.0*q2*sin(q2) - 1.0*q2^2 - 2.0))/q2^4];

C_q=[-(0.5*(2.0*l1^2*mu2*q2^3*qdot1^2 + 8.0*l1^2*mu4*q2^3*qdot1^2 + 8.0*l1^2*mu5*q2^3*qdot1^2 + 8.0*l1^2*mu6*q2^3*qdot1^2 + 8.0*l1^2*mu8*q2^3*qdot1^2 + l2^2*mu6*q1^5*qdot2^2 + 4.0*l2^2*mu8*q1^5*qdot2^2 + 0.5*l1^2*mu2*q1^2*q2^3*qdot1^2 + 2.0*l1^2*mu4*q1^2*q2^3*qdot1^2 + 2.0*l1^2*mu5*q1^2*q2^3*qdot1^2 + 2.0*l1^2*mu6*q1^2*q2^3*qdot1^2 + 2.0*l1^2*mu8*q1^2*q2^3*qdot1^2 - 2.0*l1^2*mu2*q2^3*qdot1^2*cos(q1) - 8.0*l1^2*mu4*q2^3*qdot1^2*cos(q1) - 8.0*l1^2*mu5*q2^3*qdot1^2*cos(q1) - 8.0*l1^2*mu6*q2^3*qdot1^2*cos(q1) - 8.0*l1^2*mu8*q2^3*qdot1^2*cos(q1) - 1.0*l2^2*mu6*q1^5*qdot2^2*cos(q2) - 4.0*l2^2*mu8*q1^5*qdot2^2*cos(q2) - 2.0*l1*l2*mu6*q1^3*qdot2^2 - 4.0*l1*l2*mu8*q1^3*qdot2^2 + 2.0*l2^2*mu6*q1^5*qdot1*qdot2 + 8.0*l2^2*mu8*q1^5*qdot1*qdot2 - 1.0*l1*l2*mu6*q1^3*q2^2*qdot1^2 - 2.0*l1*l2*mu8*q1^3*q2^2*qdot1^2 + 2.0*l1*l2*mu6*q1^3*qdot2^2*cos(q1) + 2.0*l1*l2*mu6*q1^3*qdot2^2*cos(q2) + 4.0*l1*l2*mu8*q1^3*qdot2^2*cos(q1) + 4.0*l1*l2*mu8*q1^3*qdot2^2*cos(q2) - 2.0*l2^2*mu6*q1^5*qdot1*qdot2*cos(q2) - 8.0*l2^2*mu8*q1^5*qdot1*qdot2*cos(q2) - 2.0*l1*l2*mu6*q1^4*qdot2^2*sin(q2) - 4.0*l1*l2*mu8*q1^4*qdot2^2*sin(q2) - 2.0*l1^2*mu2*q1*q2^3*qdot1^2*sin(q1) - 8.0*l1^2*mu4*q1*q2^3*qdot1^2*sin(q1) - 8.0*l1^2*mu5*q1*q2^3*qdot1^2*sin(q1) - 8.0*l1^2*mu6*q1*q2^3*qdot1^2*sin(q1) - 8.0*l1^2*mu8*q1*q2^3*qdot1^2*sin(q1) - 0.5*l2^2*mu6*q1^5*q2*qdot2^2*sin(q2) - 2.0*l2^2*mu8*q1^5*q2*qdot2^2*sin(q2) + 0.5*l1^2*mu2*q1^2*q2^3*qdot1^2*cos(q1) + 2.0*l1^2*mu4*q1^2*q2^3*qdot1^2*cos(q1) + 2.0*l1^2*mu5*q1^2*q2^3*qdot1^2*cos(q1) + 2.0*l1^2*mu6*q1^2*q2^3*qdot1^2*cos(q1) + 2.0*l1^2*mu8*q1^2*q2^3*qdot1^2*cos(q1) - 2.0*l1*l2*mu6*q1^3*qdot2^2*cos(q1 + q2) - 4.0*l1*l2*mu8*q1^3*qdot2^2*cos(q1 + q2) - 2.0*l1*l2*mu6*q1^3*q2*qdot2^2*sin(q1 + q2) - 4.0*l1*l2*mu8*q1^3*q2*qdot2^2*sin(q1 + q2) + 2.0*l1*l2*mu6*q1^4*q2*qdot2^2*cos(q2) + 4.0*l1*l2*mu8*q1^4*q2*qdot2^2*cos(q2) + 2.0*l1*l2*mu6*q1^3*q2*qdot2^2*sin(q2) + 4.0*l1*l2*mu8*q1^3*q2*qdot2^2*sin(q2) - 1.0*l2^2*mu6*q1^5*q2*qdot1*qdot2*sin(q2) - 4.0*l2^2*mu8*q1^5*q2*qdot1*qdot2*sin(q2) + l1*l2*mu6*q1^3*q2^2*qdot1^2*cos(q1 + q2) + l1*l2*mu6*q1^3*q2^2*qdot2^2*cos(q1 + q2) + 2.0*l1*l2*mu8*q1^3*q2^2*qdot1^2*cos(q1 + q2) + 2.0*l1*l2*mu8*q1^3*q2^2*qdot2^2*cos(q1 + q2) - 2.0*l1*l2*mu6*q1^4*q2*qdot1*qdot2 - 4.0*l1*l2*mu8*q1^4*q2*qdot1*qdot2 - 2.0*l1*l2*mu6*q1^2*q2^2*qdot1^2*sin(q1 + q2) - 4.0*l1*l2*mu8*q1^2*q2^2*qdot1^2*sin(q1 + q2) - 1.0*l1*l2*mu6*q1^3*q2^2*qdot1^2*cos(q1) + l1*l2*mu6*q1^3*q2^2*qdot1^2*cos(q2) - 1.0*l1*l2*mu6*q1^3*q2^2*qdot2^2*cos(q2) - 2.0*l1*l2*mu8*q1^3*q2^2*qdot1^2*cos(q1) + 2.0*l1*l2*mu8*q1^3*q2^2*qdot1^2*cos(q2) - 2.0*l1*l2*mu8*q1^3*q2^2*qdot2^2*cos(q2) + 2.0*l1*l2*mu6*q1^2*q2^2*qdot1^2*sin(q1) + 2.0*l1*l2*mu6*q1^2*q2^2*qdot1^2*sin(q2) + 4.0*l1*l2*mu8*q1^2*q2^2*qdot1^2*sin(q1) + 4.0*l1*l2*mu8*q1^2*q2^2*qdot1^2*sin(q2) + l1*l2*mu6*q1^4*q2^2*qdot2^2*sin(q2) + 2.0*l1*l2*mu8*q1^4*q2^2*qdot2^2*sin(q2) + 2.0*l1*l2*mu6*q1^4*q2^2*qdot1*qdot2*sin(q2) + 4.0*l1*l2*mu8*q1^4*q2^2*qdot1*qdot2*sin(q2) - 2.0*l1*l2*mu6*q1^3*q2*qdot1*qdot2*sin(q1 + q2) - 4.0*l1*l2*mu8*q1^3*q2*qdot1*qdot2*sin(q1 + q2) + 2.0*l1*l2*mu6*q1^4*q2*qdot1*qdot2*cos(q2) + 4.0*l1*l2*mu8*q1^4*q2*qdot1*qdot2*cos(q2) + 2.0*l1*l2*mu6*q1^3*q2*qdot1*qdot2*sin(q1) + 2.0*l1*l2*mu6*q1^3*q2*qdot1*qdot2*sin(q2) + 4.0*l1*l2*mu8*q1^3*q2*qdot1*qdot2*sin(q1) + 4.0*l1*l2*mu8*q1^3*q2*qdot1*qdot2*sin(q2) + 2.0*l1*l2*mu6*q1^3*q2^2*qdot1*qdot2*cos(q1 + q2) + 4.0*l1*l2*mu8*q1^3*q2^2*qdot1*qdot2*cos(q1 + q2) - 2.0*l1*l2*mu6*q1^3*q2^2*qdot1*qdot2*cos(q2) - 4.0*l1*l2*mu8*q1^3*q2^2*qdot1*qdot2*cos(q2)))/(q1^5*q2^3)
                                                                                                                                                                                                                                                                                                                                                                                                                                                                                                                                                                                                                                                                                                                                                                                                                                                                                                                                                                                                                                                                                                                                                                                                                                                                                                                                                                                                                                                                                                                                                                                                                                                                                                                                                                                                                                                                                                                                                                                                                                                                                                                                                                                                                                                     -(0.25*l2*(4.0*l2*mu6*q1^3*qdot2^2 - 4.0*l1*mu6*q2^3*qdot1^2 - 8.0*l1*mu8*q2^3*qdot1^2 + 16.0*l2*mu8*q1^3*qdot2^2 - 4.0*l1*mu6*q2^3*qdot1^2*cos(q1 + q2) - 8.0*l1*mu8*q2^3*qdot1^2*cos(q1 + q2) - 4.0*l1*mu6*q2^4*qdot1^2*sin(q1 + q2) - 8.0*l1*mu8*q2^4*qdot1^2*sin(q1 + q2) + 2.0*l1*mu6*q1^2*q2^3*qdot1^2 - 2.0*l2*mu6*q1^3*q2^2*qdot1^2 + 4.0*l1*mu8*q1^2*q2^3*qdot1^2 + l2*mu6*q1^3*q2^2*qdot2^2 - 8.0*l2*mu8*q1^3*q2^2*qdot1^2 + 4.0*l2*mu8*q1^3*q2^2*qdot2^2 + 4.0*l1*mu6*q2^3*qdot1^2*cos(q1) + 4.0*l1*mu6*q2^3*qdot1^2*cos(q2) + 8.0*l1*mu8*q2^3*qdot1^2*cos(q1) - 4.0*l2*mu6*q1^3*qdot2^2*cos(q2) + 8.0*l1*mu8*q2^3*qdot1^2*cos(q2) - 16.0*l2*mu8*q1^3*qdot2^2*cos(q2) + 4.0*l1*mu6*q2^4*qdot1^2*sin(q2) + 8.0*l1*mu8*q2^4*qdot1^2*sin(q2) + 4.0*l1*mu6*q1*q2^4*qdot1^2*cos(q2) + 8.0*l1*mu8*q1*q2^4*qdot1^2*cos(q2) - 4.0*l1*mu6*q1*q2^3*qdot1^2*sin(q2) - 8.0*l1*mu8*q1*q2^3*qdot1^2*sin(q2) - 4.0*l2*mu6*q1^3*q2*qdot2^2*sin(q2) - 16.0*l2*mu8*q1^3*q2*qdot2^2*sin(q2) - 2.0*l1*mu6*q1^2*q2^3*qdot1^2*cos(q2) + 2.0*l2*mu6*q1^3*q2^2*qdot1^2*cos(q2) - 4.0*l1*mu8*q1^2*q2^3*qdot1^2*cos(q2) + l2*mu6*q1^3*q2^2*qdot2^2*cos(q2) + 8.0*l2*mu8*q1^3*q2^2*qdot1^2*cos(q2) + 4.0*l2*mu8*q1^3*q2^2*qdot2^2*cos(q2) - 2.0*l1*mu6*q1^2*q2^4*qdot1^2*sin(q2) + l2*mu6*q1^3*q2^3*qdot1^2*sin(q2) - 4.0*l1*mu8*q1^2*q2^4*qdot1^2*sin(q2) + 4.0*l2*mu8*q1^3*q2^3*qdot1^2*sin(q2)))/(q1^3*q2^5)];
                                                                                                                                                                                                                                                                                                                                                                                                                                                                                                                                                                                                                                                                                                                                                                                                                                                                                                                                                                                                                                                                                                  
G=[-(0.005*(981.0*l2*q1^2*cos(q1 + q2)*conj(mu6) + 1962.0*l2*q1^2*cos(q1 + q2)*conj(mu8) - 981.0*l2*q1^2*conj(mu6)*cos(q1) - 1962.0*l2*q1^2*conj(mu8)*cos(q1) - 981.0*l1*mu2*q2*sin(q1) - 1962.0*l1*q2*conj(mu4)*sin(q1) - 1962.0*l1*q2*conj(mu5)*sin(q1) - 1962.0*l1*q2*conj(mu6)*sin(q1) - 1962.0*l1*q2*conj(mu8)*sin(q1) + 1962.0*l1*q1*q2*conj(mu4)*cos(q1) + 1962.0*l1*q1*q2*conj(mu5)*cos(q1) + 1962.0*l1*q1*q2*conj(mu6)*cos(q1) + 1962.0*l1*q1*q2*conj(mu8)*cos(q1) + 981.0*l1*mu2*q1*q2*cos(q1)))/(q1^2*q2)
                                                                                                                                                                                                                                                                                                                                                                                                                       -(4.905*l2*(conj(mu6) + 2.0*conj(mu8))*(sin(q1) - 1.0*sin(q1 + q2) + q2*cos(q1 + q2)))/q2^2];

K=[0.68,0;0,0.7];
D=[0.0029,0;0,0.003];

q_dotdot=(eye(2)/M)*(torque-K*[q1;q2]-D*[qdot1;qdot2]-C_q-G);
